simulink model "Basic_cosimulation_circuit"  (R2021b)
settings: Solver=ode4  StartTime=0.0  StopTime=inf  FixedStep=Ts  RelTol=1e-3  EnableMultiTasking=on
PostLoadFcn:
  | %
  | % Script for validation of swtiching model design with it's respective
  | % average model.
  | %
  | % Here it is presented the design of the inverter to the 6 kW Fuel Cell
  | % model.
  | 
  | %%% Initialization %%%
  | 
  | 
  | % ------------------------------------- %
  | % ---------- Inverter Design ---------- %
  | % ------------------------------------- %
  | 
  | %%%% Nominal Parameters %%%%
  | 
  | Pnom = 50e3;                                        % Nominal Power
  | Vdc = 400;                                          % DC Voltage - Boost
  | m = 0.6;                                            % Modulation Index
  | Vnom_peak = m*Vdc/2;                                % Peak Voltage
  | Vnom_rms = Vnom_peak/sqrt(2);                       % Rms Voltage
  | FP_min = 0.9;                                       % For Reactive Power
  |                                                     % Compensation
  | Snom = Pnom/FP_min;                                 % Apparent Power
  | Irms = Pnom/(sqrt(3)*Vnom_rms);                     % Rms Curren
  | Inom_peak = Irms*sqrt(2);                           % Peak Current
  | Zbase = Vnom_peak/Inom_peak;                        % Base Impedance
  | f = 60;                                             % Nominal Frequency
  | wnom = 2*pi*60;                                     % Angular Frequency
  | 
  | % ------------------------- %
  | % Inverter LC Filter Design %
  | % ------------------------- %
  | 
  | fsw_inv = 96*60;                                    % Switching Frequency must be a multiple of the nominal frequency
  |                                                      % for proper operation of the Artemis Block
  | ripple_inv = 0.03;
  | L_inv = ((Vdc/2)-Vnom_peak)*(1/fsw_inv)/(ripple_inv*Inom_peak);
  | 
  | % - Capacitor
  | fres = 420;                                         % Filters Ressonant Frequency
  | 
  | Cf = 1/(4*L_inv*(pi^2)*(fres^2));                % Filter Capacitor
  | Rf = 1/(wnom*Cf*50);                                % Damping Resistor
  | 
  | % --- Sample Time --- %
  | 
  | Tsw = 0.00050;
  | Ts = Tsw/10;
  | 
  | % ---------------------- %
  | % Current Control Design %
  | % ---------------------- %
  | 
  | Ron = 0.001;                                        % IGBT Resistance
  | tau_i = 1e-3;                                       % Responde Time
  | kp_current = L_inv/tau_i;                           % PI Proportional Gain
  | ki_current = (Ron)/tau_i;                           % PI Integral Gain
  | 
  | decouple = (wnom*L_inv);                            % Decoupling Gain
InitFcn:
  | %
  | % Script for validation of swtiching model design with it's respective
  | % average model.
  | %
  | % Here it is presented the design of the inverter to the 6 kW Fuel Cell
  | % model.
  | 
  | %%% Initialization %%%
  | 
  | 
  | % ------------------------------------- %
  | % ---------- Inverter Design ---------- %
  | % ------------------------------------- %
  | 
  | %%%% Nominal Parameters %%%%
  | 
  | Pnom = 50e3;                                        % Nominal Power
  | Vdc = 400;                                          % DC Voltage - Boost
  | m = 0.6;                                            % Modulation Index
  | Vnom_peak = m*Vdc/2;                                % Peak Voltage
  | Vnom_rms = Vnom_peak/sqrt(2);                       % Rms Voltage
  | FP_min = 0.9;                                       % For Reactive Power
  |                                                     % Compensation
  | Snom = Pnom/FP_min;                                 % Apparent Power
  | Irms = Pnom/(sqrt(3)*Vnom_rms);                     % Rms Curren
  | Inom_peak = Irms*sqrt(2);                           % Peak Current
  | Zbase = Vnom_peak/Inom_peak;                        % Base Impedance
  | f = 60;                                             % Nominal Frequency
  | wnom = 2*pi*60;                                     % Angular Frequency
  | 
  | % ------------------------- %
  | % Inverter LC Filter Design %
  | % ------------------------- %
  | 
  | fsw_inv = 96*60;                                    % Switching Frequency must be a multiple of the nominal frequency
  |                                                      % for proper operation of the Artemis Block
  | ripple_inv = 0.03;
  | L_inv = ((Vdc/2)-Vnom_peak)*(1/fsw_inv)/(ripple_inv*Inom_peak);
  | 
  | % - Capacitor
  | fres = 420;                                         % Filters Ressonant Frequency
  | 
  | Cf = 1/(4*L_inv*(pi^2)*(fres^2));                % Filter Capacitor
  | Rf = 1/(wnom*Cf*50);                                % Damping Resistor
  | 
  | % --- Sample Time --- %
  | 
  | Tsw = 0.00050;
  | Ts = Tsw/10;
  | 
  | % ---------------------- %
  | % Current Control Design %
  | % ---------------------- %
  | 
  | Ron = 0.001;                                        % IGBT Resistance
  | tau_i = 1e-3;                                       % Responde Time
  | kp_current = L_inv/tau_i;                           % PI Proportional Gain
  | ki_current = (Ron)/tau_i;                           % PI Integral Gain
  | 
  | decouple = (wnom*L_inv);                            % Decoupling Gain
undefined symbols (not defined in the file or in its folder): D1, Delta, DiscIntNeverNeededParam, IP, j, ph, sps, UDP
libraries: spsCurrentMeasurementLib x25, spsControlledVoltageSourceLib x21, rtlab x18, spsGroundLib x13, spsThreePhaseSeriesRLCBranchLib x13, spsControlledCurrentSourceLib x11, spsVoltageMeasurementLib x10, simulink x8, rteventslib x8, powerlib_meascontrol x7, spsThreePhaseVIMeasurementLib x4, ssn_inverter_model x4
(part 3 of 5)

== system Basic_cosimulation_circuit/SM_Master/Circuit_ITM_Source_DP_SFA/Phasor_to_Time_Domain_SFA ==
  Dynamic_Phasor : Inport
  Complex to Real-Imag4 : ComplexToRealImag
  Constant : Constant  Value=offset
  Demux : Demux  Outputs=3
  Demux1 : Demux  Outputs=2
  Gain : Gain  Gain=pi/180
  Gain3 : Gain  Gain=2*pi
  Gain4 : Gain  Gain=j*1
  Integrator : Integrator
  Magnitude-Angle to Complex : MagnitudeAngleToComplex
  Math Function : Math  SaturateOnIntegerOverflow=on
  Product : Product
  Real-Imag to Complex : RealImagToComplex
  Terminator : Terminator
  A : Outport
  B : Outport  Port=2
  C : Outport  Port=3
  wires:
  Demux/2 -> B/1
  Math Function/1 -> Product/2
  Gain4/1 -> Math Function/1
  Constant/1 -> Gain3/1
  Integrator/1 -> Gain4/1
  Dynamic_Phasor/1 -> Demux1/1
  Demux/1 -> A/1
  Product/1 -> Complex to Real-Imag4/1
  Gain3/1 -> Integrator/1
  Demux/3 -> C/1
  Complex to Real-Imag4/2 -> Terminator/1
  Complex to Real-Imag4/1 -> Demux/1
  Demux1/1 -> Real-Imag to Complex/1, Magnitude-Angle to Complex/1
  Demux1/2 -> Real-Imag to Complex/2, Gain/1
  Gain/1 -> Magnitude-Angle to Complex/2
  Real-Imag to Complex/1 -> Product/1

== system Basic_cosimulation_circuit/SM_Master/Circuit_ITM_Source_DP_SFA/Three-Phase Controlled Y-Connected Current Source ==
  Ia : Inport
  Ib : Inport  Port=2
  Ic : Inport  Port=3
  Controlled Current Source : spsControlledCurrentSourceLib/Controlled Current Source  Initialize=on  Source_Type=AC  Amplitude=0  Phase=0  Frequency=0  Measurements=None
  Controlled Current Source1 : spsControlledCurrentSourceLib/Controlled Current Source  Initialize=on  Source_Type=AC  Amplitude=0  Phase=0  Frequency=0  Measurements=None
  Controlled Current Source2 : spsControlledCurrentSourceLib/Controlled Current Source  Initialize=on  Source_Type=AC  Amplitude=0  Phase=0  Frequency=0  Measurements=None
  Ground1 : spsGroundLib/Ground  LConnTagsString=a
  A : PMIOPort  Side=Left
  B : PMIOPort  Port=2  Side=Left
  C : PMIOPort  Port=3  Side=Left
  wires:
  Ia/1 -> Controlled Current Source/1
  Ic/1 -> Controlled Current Source2/1
  Ib/1 -> Controlled Current Source1/1
  connections:
  Controlled Current Source/RConn1 -- Controlled Current Source2/RConn1 -- Ground1/LConn1 -- Controlled Current Source1/RConn1
  C/RConn1 -- Controlled Current Source2/LConn1
  B/RConn1 -- Controlled Current Source1/LConn1
  Controlled Current Source/LConn1 -- A/RConn1

== system Basic_cosimulation_circuit/SM_Master/Circuit_ITM_Source_DP_SFA/Time_Domain_To_Phasor_SFA ==
  EMT : Inport
  Complex to Magnitude-Angle : ComplexToMagnitudeAngle
  Complex to Magnitude-Angle1 : ComplexToMagnitudeAngle  Commented=on
  Complex to Real-Imag : ComplexToRealImag  Commented=on
  Complex to Real-Imag1 : ComplexToRealImag
  Constant : Constant  Value=offset
  Gain : Gain  Gain=j*(1/sqrt(3))*[0 1 -1; -1 0 1; 1 -1 0]  Multiplication=Matrix(K*u)
  Gain1 : Gain  Gain=180/pi
  Gain2 : Gain  Commented=on  Gain=j*(1/sqrt(3))*[0 1 -1; -1 0 1; 1 -1 0]  Multiplication=Matrix(K*u)
  Gain3 : Gain  Gain=-2*pi
  Gain4 : Gain  Gain=j*1
  Gain5 : Gain  Commented=on  Gain=180/pi
  Integrator : Integrator
  Math Function : Math  SaturateOnIntegerOverflow=on
  Mux1 : Mux  Inputs=2
  Mux2 : Mux  Commented=on  Inputs=2
  Mux3 : Mux  Inputs=2
  Phase/ Frequency Offset7 : commrflib2/Phase// Frequency Offset  Commented=on  phaseOffset=0  freqPort=off  freqOffset=-60
  Product : Product
  Scope : Scope
  Scope1 : Scope
  Scope2 : Scope  Commented=on  NumInputPorts=2
  Scope3 : Scope  Commented=on
  Scope4 : Scope  Commented=on
  Scope5 : Scope  Commented=on  NumInputPorts=2
  Scope6 : Scope
  Sum1 : Sum  Inputs=+|+
  Sum2 : Sum  Commented=on  Inputs=|++
  Dynamic_Phasor : Outport
  wires:
  Gain3/1 -> Integrator/1
  Sum1/1 -> Product/1
  Constant/1 -> Gain3/1
  Complex to Magnitude-Angle/1 -> Scope1/1, Mux1/1
  Gain/1 -> Sum1/1
  Gain1/1 -> Scope/1, Mux1/2
  Integrator/1 -> Gain4/1
  Math Function/1 -> Product/2
  Product/1 -> Complex to Real-Imag1/1, Complex to Magnitude-Angle/1
  Gain4/1 -> Math Function/1
  Complex to Magnitude-Angle/2 -> Gain1/1
  Gain2/1 -> Sum2/1
  Sum2/1 -> Scope2/2, Phase/ Frequency Offset7/1
  EMT/1 -> Sum1/2, Gain/1, Sum2/2, Scope2/1, Gain2/1
  Complex to Magnitude-Angle1/2 -> Gain5/1
  Phase/ Frequency Offset7/1 -> Complex to Real-Imag/1, Complex to Magnitude-Angle1/1
  Complex to Magnitude-Angle1/1 -> Scope4/1, Mux2/1
  Gain5/1 -> Scope3/1, Mux2/2
  Mux2/1 -> ?
  Complex to Real-Imag/2 -> Scope5/2
  Complex to Real-Imag/1 -> Scope5/1
  Complex to Real-Imag1/1 -> Mux3/1
  Complex to Real-Imag1/2 -> Mux3/2
  Mux3/1 -> Dynamic_Phasor/1, Scope6/1

== system Basic_cosimulation_circuit/SM_Master/Original Circuit/Control ==
  note: Control
  note: Transformation
  note: 3 Wire and PLL
  Vline : Inport
  Iabc : Inport  Port=2
  Deblock_inv : Inport  Port=3
  PQ_ref : Inport  Port=4
  Current Control : Subsystem
      settings: PortSchema="{\"entries\":[{\"content\":{\"sides\":[{\"content\":{\"connectorIds\":[\"In1\",\"In2\",\"In3\",\"In4\"]},\"type\":\"ConnectorPlacement.EquallySpacedRectSide\",\"uuid\":\"45a39461-35bf-48e0-8374-0f28be422fe8\"},{\"content\":{\"connectorIds\":[\"Out1\"],\"side\":\"RIGHT\"},\"type\":\"ConnectorPlacement.EquallySpacedRectSide\",\"uuid\":\"af171a1a-fd9b-46cd-ac56-6e4044580109\"},{\"content\":{\"connectorIds\":[\"In5\"],\"side\":\"TOP\"},\"type\":\"ConnectorPlacement.EquallySpacedRectSide\",\"uuid\":\"ea73d2ad-6043-4637-ba6c-414a87cf6777\"},{\"content\":{\"connectorIds\":[],\"side\":\"HIDDEN\"},\"type\":\"ConnectorPlacement.EquallySpacedRectSide\",\"uuid\":\"ed240fd2-007a-443e-85e9-b2acea2870c2\"}]},\"type\":\"ConnectorPlacement.EquallySpacedConnector\",\"uuid\":\"aa40401b-6e13-445e-a9b0-89ce19fbc40c\"}],\"packageUris\":[\"http://schema.mathworks.com/mf0/Connector/R2020b\"],\"version\":\"1.0\"}"
  Currents : Scope  NumInputPorts=2
  Demux : Demux  Outputs=2
  Demux1 : Demux  Outputs=2
  Meas_3_Wire : Subsystem
  Modulation : Scope
  Mux1 : Mux
  Mux2 : Mux  Inputs=2
  PQ Measure : Scope
  Park_Transformation : Subsystem
  Park_Transformation1 : Subsystem
  Power Control : Subsystem
      settings: PortSchema="{\"entries\":[{\"content\":{\"sides\":[{\"content\":{\"connectorIds\":[\"In1\"]},\"type\":\"ConnectorPlacement.EquallySpacedRectSide\",\"uuid\":\"974d39f2-3edd-4b06-9531-29f32c88933a\"},{\"content\":{\"connectorIds\":[\"Out1\"],\"side\":\"RIGHT\"},\"type\":\"ConnectorPlacement.EquallySpacedRectSide\",\"uuid\":\"24d62c8a-c61a-462a-84f0-1f0276c6dbaa\"},{\"content\":{\"connectorIds\":[],\"side\":\"TOP\"},\"type\":\"ConnectorPlacement.EquallySpacedRectSide\",\"uuid\":\"5ada6b1b-08a4-4e4d-9a20-cc19768e3a35\"},{\"content\":{\"connectorIds\":[\"In2\",\"In3\"],\"side\":\"BOTTOM\"},\"type\":\"ConnectorPlacement.EquallySpacedRectSide\",\"uuid\":\"aac35657-a4cf-4c82-a962-be637b231177\"},{\"content\":{\"connectorIds\":[],\"side\":\"HIDDEN\"},\"type\":\"ConnectorPlacement.EquallySpacedRectSide\",\"uuid\":\"6c2f95fb-9c8c-4eee-ad47-c57a643c3198\"}]},\"type\":\"ConnectorPlacement.EquallySpacedConnector\",\"uuid\":\"4f1b2c82-b884-470a-8be3-e486ca1ee764\"}],\"packageUris\":[\"http://schema.mathworks.com/mf0/Connector/R2020b\"],\"version\":\"1.0\"}"
  Power Measurement (Three-Phase) : eePowerMeasurement/Power Measurement (Three-Phase)  LabelModeActiveChoice=Continuous  F=60  K=[0 1 2 3]  Seq=Positive  Ts=0
      settings: SourceProductBaseCode=PS
  Product2 : Product
  SRF_PLL : Subsystem
  Saturation : Saturate  UpperLimit=1.1  LowerLimit=-1.1
  Terminator : Terminator
  Voltages : Scope  NumInputPorts=2
  Mabc : Outport
  Measures : Outport  Port=2
  wires:
  SRF_PLL/1(Phase) -> [phase_pll]
  Park_Transformation/1(DQ) -> Currents/2, [Idq]
  [Vabc] -> SRF_PLL/1(Vabc)
  [Vabc] -> Voltages/1, Park_Transformation1/1(ABC)
  Park_Transformation1/1(DQ) -> Voltages/2, Demux1/1, [Vdq]
  [phase_pll] -> Park_Transformation1/2(Phase)
  Saturation/1 -> Mabc/1, Modulation/1
  [dblk] -> Product2/2
  Iabc/1 -> Park_Transformation/1(ABC), Currents/1, [Iabc]
  Meas_3_Wire/1(ABC) -> [Vabc]
  Product2/1 -> Saturation/1
  Vline/1 -> Demux/1
  Demux/1 -> Meas_3_Wire/1(AB)
  Demux/2 -> Meas_3_Wire/2(BC)
  Mux1/1 -> Measures/1
  [Vdq] -> Mux1/3
  [Iabc] -> Mux1/2
  [Vabc] -> Mux1/4
  [Idq] -> Mux1/1
  Deblock_inv/1 -> [dblk], Current Control/1(Deblock)
  Current Control/1(modulation) -> Product2/1
  [Idq] -> Current Control/3(Idq)
  [Vdq] -> Current Control/4(Vdq)
  [phase_pll] -> Current Control/5(Phase)
  [phase_pll] -> Park_Transformation/2(Phase)
  Demux1/2 -> Terminator/1
  Demux1/1 -> [Vd]
  PQ_ref/1 -> Power Control/1(PQ_ref)
  [Vd] -> Power Control/2(Vd)
  [dblk] -> Power Control/3(Dblk)
  Power Control/1(Out1) -> Current Control/2(Idq_ref)
  [Vabc] -> Power Measurement (Three-Phase)/1
  [Iabc] -> Power Measurement (Three-Phase)/2
  Power Measurement (Three-Phase)/2 -> Mux2/2
  Power Measurement (Three-Phase)/1 -> Mux2/1
  Mux2/1 -> PQ Measure/1

== system Basic_cosimulation_circuit/SM_Master/Original Circuit/PWM ==
  Uabc_ref : Inport
  Constant10 : Constant  Value=2
  Constant11 : Constant  Value=fsw_inv
  Constant9 : Constant
  Demux8 : Demux  Outputs=3
  Divide7 : Product  Inputs=*/
  Divide8 : Product  Inputs=*/
  Divide9 : Product  Inputs=*/
  Mux11 : Mux  Inputs=3
  Mux12 : Mux  Inputs=2
  RTE Conversion1 : rteventslib/Signal Attributes/RTE Conversion  inputdatatype=RTE Boolean  outputdatatype=Double  compensation=Enabled  nbMaxEvents=4  sampleTime=Ts
  RTE SPWM1 : rteventslib/Sources/RTE SPWM  NumberPhases=3-ph  CenterAlignmentMode=On  MaxFreq=inf  MinFreq=0  EnablingPort=off  ComplementaryMode=on  SpaceVector=off  RiseTimeDelay=0  MaxEvents=4  SampleTime=Ts
  Scope : Scope
  Scope8 : Scope
  Selector1 : Selector  InputPortWidth=6  IndexOptions=Index vector (dialog)  Indices=[1 4 2 5 3 6]  OutputSizes=1
  Sum16 : Sum  Inputs=|++
  Sum17 : Sum  Inputs=|++
  Sum18 : Sum  Inputs=|++
  Uref : Outport  VectorParamsAs1DForOutWhenUnconnected=off
  wires:
  Uabc_ref/1 -> Demux8/1, Scope/1
  RTE SPWM1/1 -> Mux12/1
  Constant9/1 -> Sum18/2, Sum17/2, Sum16/2
  Selector1/1 -> Uref/1
  Constant11/1 -> RTE SPWM1/1
  Sum16/1 -> Divide7/1
  Constant10/1 -> Divide9/2, Divide8/2, Divide7/2
  Sum17/1 -> Divide8/1
  Divide9/1 -> Mux11/3
  RTE SPWM1/2 -> Mux12/2
  Demux8/2 -> Sum17/1
  Divide8/1 -> Mux11/2
  Sum18/1 -> Divide9/1
  Mux11/1 -> RTE SPWM1/2, Scope8/1
  Divide7/1 -> Mux11/1
  Demux8/1 -> Sum16/1
  Demux8/3 -> Sum18/1
  Mux12/1 -> RTE Conversion1/1
  RTE Conversion1/1 -> Selector1/1

== system Basic_cosimulation_circuit/SM_Master/Original_Circuit/Controllable Voltage Source  ==
  Amplitude [V] : Inport
  Phase [Deg] : Inport  Port=2
  Frequency [Hz] : Inport  Port=3
  Constant1 : Constant  Value=2*pi/3
  Controlled Voltage Source3 : spsControlledVoltageSourceLib/Controlled Voltage Source  Initialize=on  Source_Type=AC  Amplitude=0  Phase=0  Frequency=0  Measurements=None
  Controlled Voltage Source4 : spsControlledVoltageSourceLib/Controlled Voltage Source  Initialize=on  Source_Type=AC  Amplitude=0  Phase=0  Frequency=0  Measurements=None
  Controlled Voltage Source5 : spsControlledVoltageSourceLib/Controlled Voltage Source  Initialize=on  Source_Type=AC  Amplitude=0  Phase=0  Frequency=0  Measurements=None
  Cos : Trigonometry  Operator=cos
  Cos1 : Trigonometry  Operator=cos
  Cos2 : Trigonometry  Operator=cos
  Gain : Gain  Gain=2*pi
  Gain1 : Gain  Gain=pi/180
  Ground5 : spsGroundLib/Ground  LConnTagsString=a
  Integrator : Integrator  WrapState=on  WrappedStateUpperValue=2*pi  WrappedStateLowerValue=0
  Product : Product
  Product1 : Product
  Product2 : Product
  Sum : Sum  Inputs=++-
  Sum1 : Sum  Inputs=+++
  Sum2 : Sum  Inputs=|++
  A : PMIOPort  Side=Right
  B : PMIOPort  Port=2  Side=Right
  C : PMIOPort  Port=3  Side=Right
  wires:
  Sum/1 -> Cos1/1
  Amplitude [V]/1 -> Product2/1, Product1/1, Product/1
  Integrator/1 -> [phase]
  Gain/1 -> Integrator/1
  Phase [Deg]/1 -> Gain1/1
  Constant1/1 -> Sum/3, Sum1/2
  Sum2/1 -> Cos/1
  Product/1 -> Controlled Voltage Source3/1
  Cos/1 -> Product/2
  [phase] -> Sum2/1, Sum/2, Sum1/1
  Product1/1 -> Controlled Voltage Source4/1
  Product2/1 -> Controlled Voltage Source5/1
  Sum1/1 -> Cos2/1
  Cos1/1 -> Product1/2
  Cos2/1 -> Product2/2
  Frequency [Hz]/1 -> [freq_ref], Gain/1
  Gain1/1 -> Sum1/3, Sum/1, Sum2/2
  connections:
  Controlled Voltage Source4/RConn1 -- B/RConn1
  Controlled Voltage Source3/RConn1 -- A/RConn1
  Controlled Voltage Source5/RConn1 -- C/RConn1
  Controlled Voltage Source4/LConn1 -- Ground5/LConn1 -- Controlled Voltage Source5/LConn1 -- Controlled Voltage Source3/LConn1

== system Basic_cosimulation_circuit/SM_Master/VSC_ITM_Average_Moving_Window/Control ==
  note: Control
  note: Transformation
  note: 3 Wire and PLL
  Vline : Inport
  Iabc : Inport  Port=2
  Deblock_inv : Inport  Port=3
  PQ_ref : Inport  Port=4
  Current Control : Subsystem
      settings: PortSchema="{\"entries\":[{\"content\":{\"sides\":[{\"content\":{\"connectorIds\":[\"In1\",\"In2\",\"In3\",\"In4\"]},\"type\":\"ConnectorPlacement.EquallySpacedRectSide\",\"uuid\":\"45a39461-35bf-48e0-8374-0f28be422fe8\"},{\"content\":{\"connectorIds\":[\"Out1\"],\"side\":\"RIGHT\"},\"type\":\"ConnectorPlacement.EquallySpacedRectSide\",\"uuid\":\"af171a1a-fd9b-46cd-ac56-6e4044580109\"},{\"content\":{\"connectorIds\":[\"In5\"],\"side\":\"TOP\"},\"type\":\"ConnectorPlacement.EquallySpacedRectSide\",\"uuid\":\"ea73d2ad-6043-4637-ba6c-414a87cf6777\"},{\"content\":{\"connectorIds\":[],\"side\":\"HIDDEN\"},\"type\":\"ConnectorPlacement.EquallySpacedRectSide\",\"uuid\":\"ed240fd2-007a-443e-85e9-b2acea2870c2\"}]},\"type\":\"ConnectorPlacement.EquallySpacedConnector\",\"uuid\":\"aa40401b-6e13-445e-a9b0-89ce19fbc40c\"}],\"packageUris\":[\"http://schema.mathworks.com/mf0/Connector/R2020b\"],\"version\":\"1.0\"}"
  Currents : Scope  NumInputPorts=2
  Demux : Demux  Outputs=2
  Demux1 : Demux  Outputs=2
  Meas_3_Wire : Subsystem
  Modulation : Scope  Commented=on
  Mux1 : Mux  Inputs=5
  Mux2 : Mux  Inputs=2
  Park_Transformation : Subsystem
  Park_Transformation1 : Subsystem
  Power Control : Subsystem
      settings: PortSchema="{\"entries\":[{\"content\":{\"sides\":[{\"content\":{\"connectorIds\":[\"In1\"]},\"type\":\"ConnectorPlacement.EquallySpacedRectSide\",\"uuid\":\"974d39f2-3edd-4b06-9531-29f32c88933a\"},{\"content\":{\"connectorIds\":[\"Out1\"],\"side\":\"RIGHT\"},\"type\":\"ConnectorPlacement.EquallySpacedRectSide\",\"uuid\":\"24d62c8a-c61a-462a-84f0-1f0276c6dbaa\"},{\"content\":{\"connectorIds\":[],\"side\":\"TOP\"},\"type\":\"ConnectorPlacement.EquallySpacedRectSide\",\"uuid\":\"5ada6b1b-08a4-4e4d-9a20-cc19768e3a35\"},{\"content\":{\"connectorIds\":[\"In2\",\"In3\"],\"side\":\"BOTTOM\"},\"type\":\"ConnectorPlacement.EquallySpacedRectSide\",\"uuid\":\"aac35657-a4cf-4c82-a962-be637b231177\"},{\"content\":{\"connectorIds\":[],\"side\":\"HIDDEN\"},\"type\":\"ConnectorPlacement.EquallySpacedRectSide\",\"uuid\":\"6c2f95fb-9c8c-4eee-ad47-c57a643c3198\"}]},\"type\":\"ConnectorPlacement.EquallySpacedConnector\",\"uuid\":\"4f1b2c82-b884-470a-8be3-e486ca1ee764\"}],\"packageUris\":[\"http://schema.mathworks.com/mf0/Connector/R2020b\"],\"version\":\"1.0\"}"
  Power Measurement (Three-Phase) : eePowerMeasurement/Power Measurement (Three-Phase)  LabelModeActiveChoice=Discrete  F=60  K=[1]  Seq=Positive  Ts=Ts
      settings: SourceProductBaseCode=PS
  Product2 : Product
  SRF_PLL : Subsystem
  Saturation : Saturate  UpperLimit=1.1  LowerLimit=-1.1
  Terminator : Terminator
  Voltages : Scope  Commented=on  NumInputPorts=2
  Mabc : Outport
  Measures : Outport  Port=2
  Vabc : Outport  Port=3
  wires:
  SRF_PLL/1(Phase) -> [phase_pll]
  Park_Transformation/1(DQ) -> Currents/2, [Idq]
  [Vabc] -> SRF_PLL/1(Vabc)
  [Vabc] -> Voltages/1, Park_Transformation1/1(ABC)
  Park_Transformation1/1(DQ) -> Voltages/2, Demux1/1, [Vdq]
  [phase_pll] -> Park_Transformation1/2(Phase)
  Saturation/1 -> Mabc/1, Modulation/1
  [dblk] -> Product2/2
  Iabc/1 -> Park_Transformation/1(ABC), Currents/1, [Iabc]
  Meas_3_Wire/1(ABC) -> [Vabc]
  Product2/1 -> Saturation/1
  Vline/1 -> Demux/1
  Demux/1 -> Meas_3_Wire/1(AB)
  Demux/2 -> Meas_3_Wire/2(BC)
  Mux1/1 -> Measures/1
  [Vdq] -> Mux1/3
  [Iabc] -> Mux1/2
  [Vabc] -> Mux1/4, Vabc/1
  [Idq] -> Mux1/1
  Deblock_inv/1 -> [dblk], Current Control/1(Deblock)
  Current Control/1(modulation) -> Product2/1
  [Idq] -> Current Control/3(Idq)
  [Vdq] -> Current Control/4(Vdq)
  [phase_pll] -> Current Control/5(Phase)
  [phase_pll] -> Park_Transformation/2(Phase)
  Demux1/2 -> Terminator/1
  Demux1/1 -> [Vd]
  PQ_ref/1 -> Power Control/1(PQ_ref)
  [Vd] -> Power Control/2(Vd)
  [dblk] -> Power Control/3(Dblk)
  Power Control/1(Out1) -> Current Control/2(Idq_ref)
  [Vabc] -> Power Measurement (Three-Phase)/1
  [Iabc] -> Power Measurement (Three-Phase)/2
  Power Measurement (Three-Phase)/2 -> Mux2/2
  Power Measurement (Three-Phase)/1 -> Mux2/1
  Mux2/1 -> [pq_meas]
  [pq_meas] -> Mux1/5

== system Basic_cosimulation_circuit/SM_Master/VSC_ITM_Average_Moving_Window/DP - > EMT ==
  Phasor_A : Inport
  Phasor_B : Inport  Port=2
  Phasor_C : Inport  Port=3
  Demux : Demux  Outputs=2
  Demux1 : Demux  Outputs=2
  Demux2 : Demux  Outputs=2
  Subsystem : Subsystem
  Subsystem1 : Subsystem
  Subsystem2 : Subsystem
  Sinal_A : Outport
  Sinal_B : Outport  Port=2
  Sinal_C : Outport  Port=3
  wires:
  Subsystem2/1(Out1) -> Sinal_C/1
  Subsystem1/1(Out1) -> Sinal_B/1
  Subsystem/1(Out1) -> Sinal_A/1
  Demux/1 -> Subsystem/1(In1)
  Demux/2 -> Subsystem/2(Input)
  Demux1/1 -> Subsystem1/1(In1)
  Demux1/2 -> Subsystem1/2(Input1)
  Demux2/1 -> Subsystem2/1(In1)
  Demux2/2 -> Subsystem2/2(Input2)
  Phasor_A/1 -> Demux/1
  Phasor_B/1 -> Demux1/1
  Phasor_C/1 -> Demux2/1

== system Basic_cosimulation_circuit/SM_Master/VSC_ITM_Average_Moving_Window/Dynamic Phasor coeficientes extraction ==
  EMT_Signal : Inport
  Demux : Demux  Outputs=3
  Fourier_A : powerlib_meascontrol/Measurements/Fourier  Freq=60  n=1  InInit=[1,0]  Ts=Ts
  Fourier_B : powerlib_meascontrol/Measurements/Fourier  Freq=60  n=1  InInit=[1,-120 ]  Ts=Ts
  Fourier_C : powerlib_meascontrol/Measurements/Fourier  Freq=60  n=1  InInit=[1,+120 ]  Ts=Ts
  Mux : Mux  Inputs=2
  Mux1 : Mux  Inputs=2
  Mux2 : Mux  Inputs=2
  deg->rad : Gain  Gain=pi/180  SaturateOnIntegerOverflow=on  OutDataTypeStr=Inherit: Same as input  ParamDataTypeStr=Inherit: Same as input
  deg->rad1 : Gain  Gain=pi/180  SaturateOnIntegerOverflow=on  OutDataTypeStr=Inherit: Same as input  ParamDataTypeStr=Inherit: Same as input
  deg->rad2 : Gain  Gain=pi/180  SaturateOnIntegerOverflow=on  OutDataTypeStr=Inherit: Same as input  ParamDataTypeStr=Inherit: Same as input
  Phasor_A : Outport
  Phasor_B : Outport  Port=2
  Phasor_C : Outport  Port=3
  wires:
  Demux/2 -> Fourier_B/1
  deg->rad1/1 -> Mux2/2
  Demux/3 -> Fourier_C/1
  Demux/1 -> Fourier_A/1
  Fourier_C/1 -> Mux1/1
  EMT_Signal/1 -> Demux/1
  Fourier_B/2 -> deg->rad1/1
  deg->rad2/1 -> Mux1/2
  Fourier_A/2 -> deg->rad/1
  Fourier_C/2 -> deg->rad2/1
  Fourier_A/1 -> Mux/1
  deg->rad/1 -> Mux/2
  Fourier_B/1 -> Mux2/1
  Mux/1 -> Phasor_A/1
  Mux2/1 -> Phasor_B/1
  Mux1/1 -> Phasor_C/1

== system Basic_cosimulation_circuit/SM_Master/VSC_ITM_Average_Moving_Window/PWM ==
  Uabc_ref : Inport
  Constant10 : Constant  Value=2
  Constant11 : Constant  Value=fsw_inv
  Constant9 : Constant
  Demux8 : Demux  Outputs=3
  Divide7 : Product  Inputs=*/
  Divide8 : Product  Inputs=*/
  Divide9 : Product  Inputs=*/
  Mux11 : Mux  Inputs=3
  Mux12 : Mux  Inputs=2
  RTE Conversion1 : rteventslib/Signal Attributes/RTE Conversion  inputdatatype=RTE Boolean  outputdatatype=Double  compensation=Enabled  nbMaxEvents=4  sampleTime=Ts
  RTE SPWM1 : rteventslib/Sources/RTE SPWM  NumberPhases=3-ph  CenterAlignmentMode=On  MaxFreq=inf  MinFreq=0  EnablingPort=off  ComplementaryMode=on  SpaceVector=off  RiseTimeDelay=0  MaxEvents=4  SampleTime=Ts
  Scope : Scope
  Scope8 : Scope
  Selector1 : Selector  InputPortWidth=6  IndexOptions=Index vector (dialog)  Indices=[1 4 2 5 3 6]  OutputSizes=1
  Sum16 : Sum  Inputs=|++
  Sum17 : Sum  Inputs=|++
  Sum18 : Sum  Inputs=|++
  Uref : Outport  VectorParamsAs1DForOutWhenUnconnected=off
  wires:
  Uabc_ref/1 -> Demux8/1, Scope/1
  RTE SPWM1/1 -> Mux12/1
  Constant9/1 -> Sum18/2, Sum17/2, Sum16/2
  Selector1/1 -> Uref/1
  Constant11/1 -> RTE SPWM1/1
  Sum16/1 -> Divide7/1
  Constant10/1 -> Divide9/2, Divide8/2, Divide7/2
  Sum17/1 -> Divide8/1
  Divide9/1 -> Mux11/3
  RTE SPWM1/2 -> Mux12/2
  Demux8/2 -> Sum17/1
  Divide8/1 -> Mux11/2
  Sum18/1 -> Divide9/1
  Mux11/1 -> RTE SPWM1/2, Scope8/1
  Divide7/1 -> Mux11/1
  Demux8/1 -> Sum16/1
  Demux8/3 -> Sum18/1
  Mux12/1 -> RTE Conversion1/1
  RTE Conversion1/1 -> Selector1/1

== system Basic_cosimulation_circuit/SM_Master/VSC_ITM_Average_Moving_Window/Three-Phase Controlled Y-Connected Voltage Source  ==
  Va : Inport
  Vb : Inport  Port=2
  Vc : Inport  Port=3
  Controlled Voltage Source : spsControlledVoltageSourceLib/Controlled Voltage Source  Initialize=off  Source_Type=AC  Amplitude=0  Phase=0  Frequency=0  Measurements=None
  Controlled Voltage Source1 : spsControlledVoltageSourceLib/Controlled Voltage Source  Initialize=off  Source_Type=AC  Amplitude=0  Phase=0  Frequency=0  Measurements=None
  Controlled Voltage Source2 : spsControlledVoltageSourceLib/Controlled Voltage Source  Initialize=off  Source_Type=AC  Amplitude=0  Phase=0  Frequency=0  Measurements=None
  Ground : spsGroundLib/Ground  LConnTagsString=a
  + : PMIOPort  Side=Right
  +1 : PMIOPort  Port=2  Side=Right
  +2 : PMIOPort  Port=3  Side=Right
  wires:
  Vb/1 -> Controlled Voltage Source1/1
  Va/1 -> Controlled Voltage Source/1
  Vc/1 -> Controlled Voltage Source2/1
  connections:
  Controlled Voltage Source/RConn1 -- +/RConn1
  Controlled Voltage Source1/RConn1 -- +1/RConn1
  Controlled Voltage Source2/RConn1 -- +2/RConn1
  Controlled Voltage Source2/LConn1 -- Controlled Voltage Source/LConn1 -- Controlled Voltage Source1/LConn1 -- Ground/LConn1

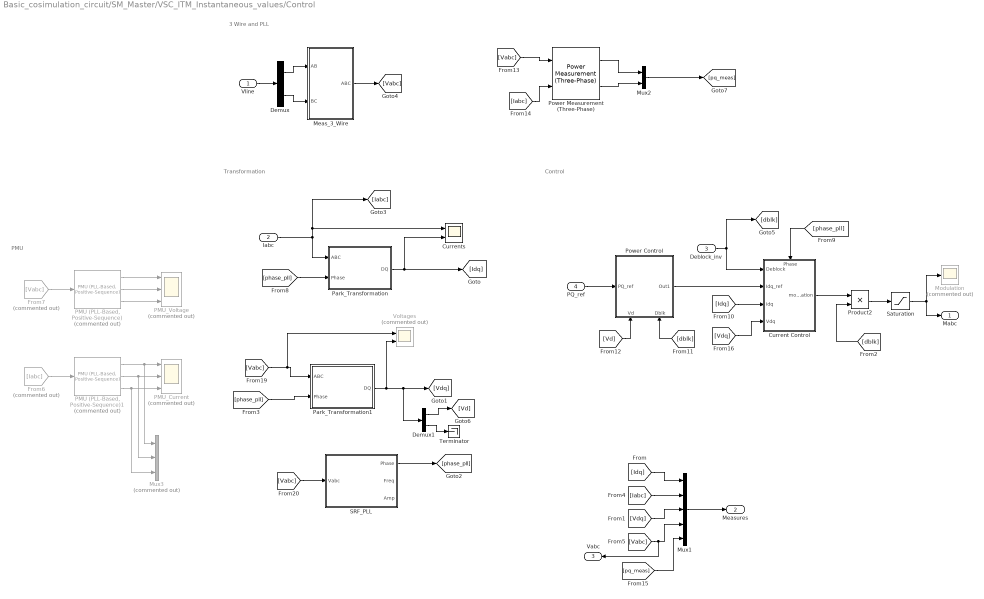
== system Basic_cosimulation_circuit/SM_Master/VSC_ITM_Instantaneous_values/Control ==
  note: PMU
  note: Control
  note: Transformation
  note: 3 Wire and PLL
  Vline : Inport
  Iabc : Inport  Port=2
  Deblock_inv : Inport  Port=3
  PQ_ref : Inport  Port=4
  Current Control : Subsystem
      settings: PortSchema="{\"entries\":[{\"content\":{\"sides\":[{\"content\":{\"connectorIds\":[\"In1\",\"In2\",\"In3\",\"In4\"]},\"type\":\"ConnectorPlacement.EquallySpacedRectSide\",\"uuid\":\"45a39461-35bf-48e0-8374-0f28be422fe8\"},{\"content\":{\"connectorIds\":[\"Out1\"],\"side\":\"RIGHT\"},\"type\":\"ConnectorPlacement.EquallySpacedRectSide\",\"uuid\":\"af171a1a-fd9b-46cd-ac56-6e4044580109\"},{\"content\":{\"connectorIds\":[\"In5\"],\"side\":\"TOP\"},\"type\":\"ConnectorPlacement.EquallySpacedRectSide\",\"uuid\":\"ea73d2ad-6043-4637-ba6c-414a87cf6777\"},{\"content\":{\"connectorIds\":[],\"side\":\"HIDDEN\"},\"type\":\"ConnectorPlacement.EquallySpacedRectSide\",\"uuid\":\"ed240fd2-007a-443e-85e9-b2acea2870c2\"}]},\"type\":\"ConnectorPlacement.EquallySpacedConnector\",\"uuid\":\"aa40401b-6e13-445e-a9b0-89ce19fbc40c\"}],\"packageUris\":[\"http://schema.mathworks.com/mf0/Connector/R2020b\"],\"version\":\"1.0\"}"
  Currents : Scope  NumInputPorts=2
  Demux : Demux  Outputs=2
  Demux1 : Demux  Outputs=2
  From6 : From  Commented=on  GotoTag=Iabc
  From7 : From  Commented=on  GotoTag=Vabc
  Meas_3_Wire : Subsystem
  Modulation : Scope  Commented=on
  Mux1 : Mux  Inputs=5
  Mux2 : Mux  Inputs=2
  Mux3 : Mux  Commented=on  Inputs=3
  "PMU (PLL-Based, Positive-Sequence)" : powerlib_meascontrol/Measurements/PMU (PLL-Based, Positive-Sequence)  Commented=on  nominalFrequency=60  samplingRate=48  reportingFactor=1
      settings: SourceProductBaseCode=PS
  "PMU (PLL-Based, Positive-Sequence)1" : powerlib_meascontrol/Measurements/PMU (PLL-Based, Positive-Sequence)  Commented=on  nominalFrequency=60  samplingRate=48  reportingFactor=1
      settings: SourceProductBaseCode=PS
  PMU_Current : Scope  Commented=on  NumInputPorts=3
  PMU_Voltage : Scope  Commented=on  NumInputPorts=3
  Park_Transformation : Subsystem
  Park_Transformation1 : Subsystem
  Power Control : Subsystem
      settings: PortSchema="{\"entries\":[{\"content\":{\"sides\":[{\"content\":{\"connectorIds\":[\"In1\"]},\"type\":\"ConnectorPlacement.EquallySpacedRectSide\",\"uuid\":\"974d39f2-3edd-4b06-9531-29f32c88933a\"},{\"content\":{\"connectorIds\":[\"Out1\"],\"side\":\"RIGHT\"},\"type\":\"ConnectorPlacement.EquallySpacedRectSide\",\"uuid\":\"24d62c8a-c61a-462a-84f0-1f0276c6dbaa\"},{\"content\":{\"connectorIds\":[],\"side\":\"TOP\"},\"type\":\"ConnectorPlacement.EquallySpacedRectSide\",\"uuid\":\"5ada6b1b-08a4-4e4d-9a20-cc19768e3a35\"},{\"content\":{\"connectorIds\":[\"In2\",\"In3\"],\"side\":\"BOTTOM\"},\"type\":\"ConnectorPlacement.EquallySpacedRectSide\",\"uuid\":\"aac35657-a4cf-4c82-a962-be637b231177\"},{\"content\":{\"connectorIds\":[],\"side\":\"HIDDEN\"},\"type\":\"ConnectorPlacement.EquallySpacedRectSide\",\"uuid\":\"6c2f95fb-9c8c-4eee-ad47-c57a643c3198\"}]},\"type\":\"ConnectorPlacement.EquallySpacedConnector\",\"uuid\":\"4f1b2c82-b884-470a-8be3-e486ca1ee764\"}],\"packageUris\":[\"http://schema.mathworks.com/mf0/Connector/R2020b\"],\"version\":\"1.0\"}"
  Power Measurement (Three-Phase) : eePowerMeasurement/Power Measurement (Three-Phase)  LabelModeActiveChoice=Discrete  F=60  K=[1]  Seq=Positive  Ts=Ts
      settings: SourceProductBaseCode=PS
  Product2 : Product
  SRF_PLL : Subsystem
  Saturation : Saturate  UpperLimit=1.1  LowerLimit=-1.1
  Terminator : Terminator
  Voltages : Scope  Commented=on  NumInputPorts=2
  Mabc : Outport
  Measures : Outport  Port=2
  Vabc : Outport  Port=3
  wires:
  SRF_PLL/1(Phase) -> [phase_pll]
  Park_Transformation/1(DQ) -> Currents/2, [Idq]
  [Vabc] -> SRF_PLL/1(Vabc)
  [Vabc] -> Voltages/1, Park_Transformation1/1(ABC)
  Park_Transformation1/1(DQ) -> Voltages/2, Demux1/1, [Vdq]
  [phase_pll] -> Park_Transformation1/2(Phase)
  Saturation/1 -> Mabc/1, Modulation/1
  [dblk] -> Product2/2
  Iabc/1 -> Park_Transformation/1(ABC), Currents/1, [Iabc]
  Meas_3_Wire/1(ABC) -> [Vabc]
  Product2/1 -> Saturation/1
  Vline/1 -> Demux/1
  Demux/1 -> Meas_3_Wire/1(AB)
  Demux/2 -> Meas_3_Wire/2(BC)
  Mux1/1 -> Measures/1
  [Vdq] -> Mux1/3
  [Iabc] -> Mux1/2
  [Vabc] -> Mux1/4, Vabc/1
  [Idq] -> Mux1/1
  From7/1 -> "PMU (PLL-Based, Positive-Sequence)"/1
  From6/1 -> "PMU (PLL-Based, Positive-Sequence)1"/1
  "PMU (PLL-Based, Positive-Sequence)"/1 -> PMU_Voltage/1
  "PMU (PLL-Based, Positive-Sequence)"/2 -> PMU_Voltage/2
  "PMU (PLL-Based, Positive-Sequence)"/3 -> PMU_Voltage/3
  "PMU (PLL-Based, Positive-Sequence)1"/1 -> Mux3/1, PMU_Current/1
  "PMU (PLL-Based, Positive-Sequence)1"/2 -> Mux3/2, PMU_Current/2
  "PMU (PLL-Based, Positive-Sequence)1"/3 -> Mux3/3, PMU_Current/3
  Deblock_inv/1 -> [dblk], Current Control/1(Deblock)
  Current Control/1(modulation) -> Product2/1
  [Idq] -> Current Control/3(Idq)
  [Vdq] -> Current Control/4(Vdq)
  [phase_pll] -> Current Control/5(Phase)
  [phase_pll] -> Park_Transformation/2(Phase)
  Demux1/2 -> Terminator/1
  Demux1/1 -> [Vd]
  PQ_ref/1 -> Power Control/1(PQ_ref)
  [Vd] -> Power Control/2(Vd)
  [dblk] -> Power Control/3(Dblk)
  Power Control/1(Out1) -> Current Control/2(Idq_ref)
  [Vabc] -> Power Measurement (Three-Phase)/1
  [Iabc] -> Power Measurement (Three-Phase)/2
  Power Measurement (Three-Phase)/2 -> Mux2/2
  Power Measurement (Three-Phase)/1 -> Mux2/1
  Mux2/1 -> [pq_meas]
  [pq_meas] -> Mux1/5

== system Basic_cosimulation_circuit/SM_Master/VSC_ITM_Instantaneous_values/PWM ==
  Uabc_ref : Inport
  Constant10 : Constant  Value=2
  Constant11 : Constant  Value=fsw_inv
  Constant9 : Constant
  Demux8 : Demux  Outputs=3
  Divide7 : Product  Inputs=*/
  Divide8 : Product  Inputs=*/
  Divide9 : Product  Inputs=*/
  Mux11 : Mux  Inputs=3
  Mux12 : Mux  Inputs=2
  RTE Conversion1 : rteventslib/Signal Attributes/RTE Conversion  inputdatatype=RTE Boolean  outputdatatype=Double  compensation=Enabled  nbMaxEvents=4  sampleTime=Ts
  RTE SPWM1 : rteventslib/Sources/RTE SPWM  NumberPhases=3-ph  CenterAlignmentMode=On  MaxFreq=inf  MinFreq=0  EnablingPort=off  ComplementaryMode=on  SpaceVector=off  RiseTimeDelay=0  MaxEvents=4  SampleTime=Ts
  Scope : Scope
  Scope8 : Scope
  Selector1 : Selector  InputPortWidth=6  IndexOptions=Index vector (dialog)  Indices=[1 4 2 5 3 6]  OutputSizes=1
  Sum16 : Sum  Inputs=|++
  Sum17 : Sum  Inputs=|++
  Sum18 : Sum  Inputs=|++
  Uref : Outport  VectorParamsAs1DForOutWhenUnconnected=off
  wires:
  Uabc_ref/1 -> Demux8/1, Scope/1
  RTE SPWM1/1 -> Mux12/1
  Constant9/1 -> Sum18/2, Sum17/2, Sum16/2
  Selector1/1 -> Uref/1
  Constant11/1 -> RTE SPWM1/1
  Sum16/1 -> Divide7/1
  Constant10/1 -> Divide9/2, Divide8/2, Divide7/2
  Sum17/1 -> Divide8/1
  Divide9/1 -> Mux11/3
  RTE SPWM1/2 -> Mux12/2
  Demux8/2 -> Sum17/1
  Divide8/1 -> Mux11/2
  Sum18/1 -> Divide9/1
  Mux11/1 -> RTE SPWM1/2, Scope8/1
  Divide7/1 -> Mux11/1
  Demux8/1 -> Sum16/1
  Demux8/3 -> Sum18/1
  Mux12/1 -> RTE Conversion1/1
  RTE Conversion1/1 -> Selector1/1

== system Basic_cosimulation_circuit/SM_Master/VSC_ITM_Instantaneous_values/Three-Phase Controlled Y-Connected Voltage Source  ==
  Va : Inport
  Vb : Inport  Port=2
  Vc : Inport  Port=3
  Controlled Voltage Source : spsControlledVoltageSourceLib/Controlled Voltage Source  Initialize=off  Source_Type=AC  Amplitude=0  Phase=0  Frequency=0  Measurements=None
  Controlled Voltage Source1 : spsControlledVoltageSourceLib/Controlled Voltage Source  Initialize=off  Source_Type=AC  Amplitude=0  Phase=0  Frequency=0  Measurements=None
  Controlled Voltage Source2 : spsControlledVoltageSourceLib/Controlled Voltage Source  Initialize=off  Source_Type=AC  Amplitude=0  Phase=0  Frequency=0  Measurements=None
  Ground : spsGroundLib/Ground  LConnTagsString=a
  + : PMIOPort  Side=Right
  +1 : PMIOPort  Port=2  Side=Right
  +2 : PMIOPort  Port=3  Side=Right
  wires:
  Vb/1 -> Controlled Voltage Source1/1
  Va/1 -> Controlled Voltage Source/1
  Vc/1 -> Controlled Voltage Source2/1
  connections:
  Controlled Voltage Source/RConn1 -- +/RConn1
  Controlled Voltage Source1/RConn1 -- +1/RConn1
  Controlled Voltage Source2/RConn1 -- +2/RConn1
  Controlled Voltage Source2/LConn1 -- Controlled Voltage Source/LConn1 -- Controlled Voltage Source1/LConn1 -- Ground/LConn1

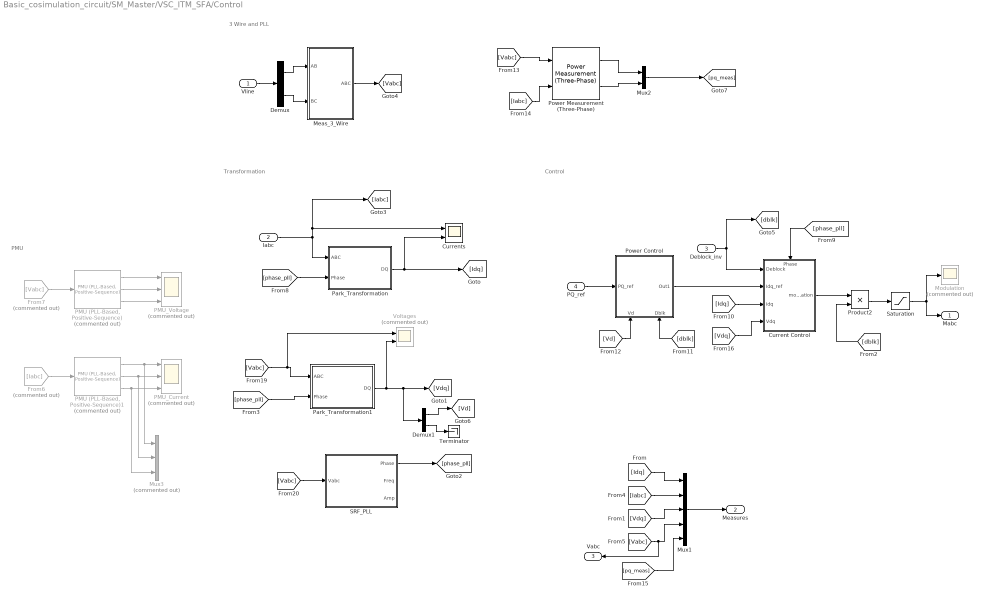
== system Basic_cosimulation_circuit/SM_Master/VSC_ITM_SFA/Control ==
  note: PMU
  note: Control
  note: Transformation
  note: 3 Wire and PLL
  Vline : Inport
  Iabc : Inport  Port=2
  Deblock_inv : Inport  Port=3
  PQ_ref : Inport  Port=4
  Current Control : Subsystem
      settings: PortSchema="{\"entries\":[{\"content\":{\"sides\":[{\"content\":{\"connectorIds\":[\"In1\",\"In2\",\"In3\",\"In4\"]},\"type\":\"ConnectorPlacement.EquallySpacedRectSide\",\"uuid\":\"45a39461-35bf-48e0-8374-0f28be422fe8\"},{\"content\":{\"connectorIds\":[\"Out1\"],\"side\":\"RIGHT\"},\"type\":\"ConnectorPlacement.EquallySpacedRectSide\",\"uuid\":\"af171a1a-fd9b-46cd-ac56-6e4044580109\"},{\"content\":{\"connectorIds\":[\"In5\"],\"side\":\"TOP\"},\"type\":\"ConnectorPlacement.EquallySpacedRectSide\",\"uuid\":\"ea73d2ad-6043-4637-ba6c-414a87cf6777\"},{\"content\":{\"connectorIds\":[],\"side\":\"HIDDEN\"},\"type\":\"ConnectorPlacement.EquallySpacedRectSide\",\"uuid\":\"ed240fd2-007a-443e-85e9-b2acea2870c2\"}]},\"type\":\"ConnectorPlacement.EquallySpacedConnector\",\"uuid\":\"aa40401b-6e13-445e-a9b0-89ce19fbc40c\"}],\"packageUris\":[\"http://schema.mathworks.com/mf0/Connector/R2020b\"],\"version\":\"1.0\"}"
  Currents : Scope  NumInputPorts=2
  Demux : Demux  Outputs=2
  Demux1 : Demux  Outputs=2
  From6 : From  Commented=on  GotoTag=Iabc
  From7 : From  Commented=on  GotoTag=Vabc
  Meas_3_Wire : Subsystem
  Modulation : Scope  Commented=on
  Mux1 : Mux  Inputs=5
  Mux2 : Mux  Inputs=2
  Mux3 : Mux  Commented=on  Inputs=3
  "PMU (PLL-Based, Positive-Sequence)" : spsPMUPLLBasedPositiveSequenceLib/PMU (PLL-Based, Positive-Sequence)  Commented=on  nominalFrequency=60  samplingRate=48  reportingFactor=1
      settings: SourceProductBaseCode=PS
  "PMU (PLL-Based, Positive-Sequence)1" : spsPMUPLLBasedPositiveSequenceLib/PMU (PLL-Based, Positive-Sequence)  Commented=on  nominalFrequency=60  samplingRate=48  reportingFactor=1
      settings: SourceProductBaseCode=PS
  PMU_Current : Scope  Commented=on  NumInputPorts=3
  PMU_Voltage : Scope  Commented=on  NumInputPorts=3
  Park_Transformation : Subsystem
  Park_Transformation1 : Subsystem
  Power Control : Subsystem
      settings: PortSchema="{\"entries\":[{\"content\":{\"sides\":[{\"content\":{\"connectorIds\":[\"In1\"]},\"type\":\"ConnectorPlacement.EquallySpacedRectSide\",\"uuid\":\"974d39f2-3edd-4b06-9531-29f32c88933a\"},{\"content\":{\"connectorIds\":[\"Out1\"],\"side\":\"RIGHT\"},\"type\":\"ConnectorPlacement.EquallySpacedRectSide\",\"uuid\":\"24d62c8a-c61a-462a-84f0-1f0276c6dbaa\"},{\"content\":{\"connectorIds\":[],\"side\":\"TOP\"},\"type\":\"ConnectorPlacement.EquallySpacedRectSide\",\"uuid\":\"5ada6b1b-08a4-4e4d-9a20-cc19768e3a35\"},{\"content\":{\"connectorIds\":[\"In2\",\"In3\"],\"side\":\"BOTTOM\"},\"type\":\"ConnectorPlacement.EquallySpacedRectSide\",\"uuid\":\"aac35657-a4cf-4c82-a962-be637b231177\"},{\"content\":{\"connectorIds\":[],\"side\":\"HIDDEN\"},\"type\":\"ConnectorPlacement.EquallySpacedRectSide\",\"uuid\":\"6c2f95fb-9c8c-4eee-ad47-c57a643c3198\"}]},\"type\":\"ConnectorPlacement.EquallySpacedConnector\",\"uuid\":\"4f1b2c82-b884-470a-8be3-e486ca1ee764\"}],\"packageUris\":[\"http://schema.mathworks.com/mf0/Connector/R2020b\"],\"version\":\"1.0\"}"
  Power Measurement (Three-Phase) : eePowerMeasurement/Power Measurement (Three-Phase)  LabelModeActiveChoice=Discrete  F=60  K=[1]  Seq=Positive  Ts=Ts
      settings: SourceProductBaseCode=PS
  Product2 : Product
  SRF_PLL : Subsystem
  Saturation : Saturate  UpperLimit=1.1  LowerLimit=-1.1
  Terminator : Terminator
  Voltages : Scope  Commented=on  NumInputPorts=2
  Mabc : Outport
  Measures : Outport  Port=2
  Vabc : Outport  Port=3
  wires:
  SRF_PLL/1(Phase) -> [phase_pll]
  Park_Transformation/1(DQ) -> Currents/2, [Idq]
  [Vabc] -> SRF_PLL/1(Vabc)
  [Vabc] -> Voltages/1, Park_Transformation1/1(ABC)
  Park_Transformation1/1(DQ) -> Voltages/2, Demux1/1, [Vdq]
  [phase_pll] -> Park_Transformation1/2(Phase)
  Saturation/1 -> Mabc/1, Modulation/1
  [dblk] -> Product2/2
  Iabc/1 -> Park_Transformation/1(ABC), Currents/1, [Iabc]
  Meas_3_Wire/1(ABC) -> [Vabc]
  Product2/1 -> Saturation/1
  Vline/1 -> Demux/1
  Demux/1 -> Meas_3_Wire/1(AB)
  Demux/2 -> Meas_3_Wire/2(BC)
  Mux1/1 -> Measures/1
  [Vdq] -> Mux1/3
  [Iabc] -> Mux1/2
  [Vabc] -> Mux1/4, Vabc/1
  [Idq] -> Mux1/1
  From7/1 -> "PMU (PLL-Based, Positive-Sequence)"/1
  From6/1 -> "PMU (PLL-Based, Positive-Sequence)1"/1
  "PMU (PLL-Based, Positive-Sequence)"/1 -> PMU_Voltage/1
  "PMU (PLL-Based, Positive-Sequence)"/2 -> PMU_Voltage/2
  "PMU (PLL-Based, Positive-Sequence)"/3 -> PMU_Voltage/3
  "PMU (PLL-Based, Positive-Sequence)1"/1 -> Mux3/1, PMU_Current/1
  "PMU (PLL-Based, Positive-Sequence)1"/2 -> Mux3/2, PMU_Current/2
  "PMU (PLL-Based, Positive-Sequence)1"/3 -> Mux3/3, PMU_Current/3
  Deblock_inv/1 -> [dblk], Current Control/1(Deblock)
  Current Control/1(modulation) -> Product2/1
  [Idq] -> Current Control/3(Idq)
  [Vdq] -> Current Control/4(Vdq)
  [phase_pll] -> Current Control/5(Phase)
  [phase_pll] -> Park_Transformation/2(Phase)
  Demux1/2 -> Terminator/1
  Demux1/1 -> [Vd]
  PQ_ref/1 -> Power Control/1(PQ_ref)
  [Vd] -> Power Control/2(Vd)
  [dblk] -> Power Control/3(Dblk)
  Power Control/1(Out1) -> Current Control/2(Idq_ref)
  [Vabc] -> Power Measurement (Three-Phase)/1
  [Iabc] -> Power Measurement (Three-Phase)/2
  Power Measurement (Three-Phase)/2 -> Mux2/2
  Power Measurement (Three-Phase)/1 -> Mux2/1
  Mux2/1 -> [pq_meas]
  [pq_meas] -> Mux1/5

== system Basic_cosimulation_circuit/SM_Master/VSC_ITM_SFA/PWM ==
  Uabc_ref : Inport
  Constant10 : Constant  Value=2
  Constant11 : Constant  Value=fsw_inv
  Constant9 : Constant
  Demux8 : Demux  Outputs=3
  Divide7 : Product  Inputs=*/
  Divide8 : Product  Inputs=*/
  Divide9 : Product  Inputs=*/
  Mux11 : Mux  Inputs=3
  Mux12 : Mux  Inputs=2
  RTE Conversion1 : rteventslib/Signal Attributes/RTE Conversion  inputdatatype=RTE Boolean  outputdatatype=Double  compensation=Enabled  nbMaxEvents=4  sampleTime=Ts
  RTE SPWM1 : rteventslib/Sources/RTE SPWM  NumberPhases=3-ph  CenterAlignmentMode=On  MaxFreq=inf  MinFreq=0  EnablingPort=off  ComplementaryMode=on  SpaceVector=off  RiseTimeDelay=0  MaxEvents=4  SampleTime=Ts
  Scope : Scope
  Scope8 : Scope
  Selector1 : Selector  InputPortWidth=6  IndexOptions=Index vector (dialog)  Indices=[1 4 2 5 3 6]  OutputSizes=1
  Sum16 : Sum  Inputs=|++
  Sum17 : Sum  Inputs=|++
  Sum18 : Sum  Inputs=|++
  Uref : Outport  VectorParamsAs1DForOutWhenUnconnected=off
  wires:
  Uabc_ref/1 -> Demux8/1, Scope/1
  RTE SPWM1/1 -> Mux12/1
  Constant9/1 -> Sum18/2, Sum17/2, Sum16/2
  Selector1/1 -> Uref/1
  Constant11/1 -> RTE SPWM1/1
  Sum16/1 -> Divide7/1
  Constant10/1 -> Divide9/2, Divide8/2, Divide7/2
  Sum17/1 -> Divide8/1
  Divide9/1 -> Mux11/3
  RTE SPWM1/2 -> Mux12/2
  Demux8/2 -> Sum17/1
  Divide8/1 -> Mux11/2
  Sum18/1 -> Divide9/1
  Mux11/1 -> RTE SPWM1/2, Scope8/1
  Divide7/1 -> Mux11/1
  Demux8/1 -> Sum16/1
  Demux8/3 -> Sum18/1
  Mux12/1 -> RTE Conversion1/1
  RTE Conversion1/1 -> Selector1/1

== system Basic_cosimulation_circuit/SM_Master/VSC_ITM_SFA/Phasor_to_Time_Domain_SFA ==
  Dynamic_Phasor : Inport
  Complex to Real-Imag4 : ComplexToRealImag
  Constant : Constant  Value=offset
  Deg->Rad : Gain  Gain=pi/180
  Demux1 : Demux  Outputs=2
  Gain3 : Gain  Gain=2*pi
  Gain4 : Gain  Gain=j*1
  Integrator with Wrapped State (Discrete or Continuous) : eeGeneralControl/Integrator with Wrapped State (Discrete or Continuous)  LabelModeActiveChoice=Discrete  WrappedStateUpperValue=2*pi  WrappedStateLowerValue=0  x0=0  Ts=-1
      settings: SourceProductBaseCode=PS
  Magnitude-Angle to Complex : MagnitudeAngleToComplex
  Math Function : Math  SaturateOnIntegerOverflow=on
  Product : Product
  Terminator : Terminator
  EMT : Outport
  wires:
  Dynamic_Phasor/1 -> Demux1/1
  Product/1 -> Complex to Real-Imag4/1  "Analytic Signal"
  Magnitude-Angle to Complex/1 -> Product/1  "Dynamic Phasor"
  Complex to Real-Imag4/2 -> Terminator/1
  Complex to Real-Imag4/1 -> EMT/1
  Demux1/1 -> Magnitude-Angle to Complex/1
  Demux1/2 -> Deg->Rad/1
  Deg->Rad/1 -> Magnitude-Angle to Complex/2
  Constant/1 -> Gain3/1
  Math Function/1 -> Product/2  "Phase Shift"
  Gain4/1 -> Math Function/1
  Gain3/1 -> Integrator with Wrapped State (Discrete or Continuous)/1
  Integrator with Wrapped State (Discrete or Continuous)/1 -> Gain4/1

== system Basic_cosimulation_circuit/SM_Master/VSC_ITM_SFA/Three-Phase Controlled Y-Connected Voltage Source  ==
  Va : Inport
  Vb : Inport  Port=2
  Vc : Inport  Port=3
  Controlled Voltage Source : spsControlledVoltageSourceLib/Controlled Voltage Source  Initialize=on  Source_Type=AC  Amplitude=0  Phase=0  Frequency=0  Measurements=None
  Controlled Voltage Source1 : spsControlledVoltageSourceLib/Controlled Voltage Source  Initialize=on  Source_Type=AC  Amplitude=0  Phase=0  Frequency=0  Measurements=None
  Controlled Voltage Source2 : spsControlledVoltageSourceLib/Controlled Voltage Source  Initialize=on  Source_Type=AC  Amplitude=0  Phase=0  Frequency=0  Measurements=None
  Ground : spsGroundLib/Ground  LConnTagsString=a
  A : PMIOPort  Side=Right
  B : PMIOPort  Port=2  Side=Right
  C : PMIOPort  Port=3  Side=Right
  wires:
  Vb/1 -> Controlled Voltage Source1/1
  Va/1 -> Controlled Voltage Source/1
  Vc/1 -> Controlled Voltage Source2/1
  connections:
  Controlled Voltage Source/RConn1 -- A/RConn1
  Controlled Voltage Source1/RConn1 -- B/RConn1
  Controlled Voltage Source2/RConn1 -- C/RConn1
  Controlled Voltage Source2/LConn1 -- Controlled Voltage Source/LConn1 -- Controlled Voltage Source1/LConn1 -- Ground/LConn1

== system Basic_cosimulation_circuit/SM_Master/VSC_ITM_SFA/Time_Domain_To_Phasor_SFA ==
  EMT : Inport
  Complex to Magnitude-Angle : ComplexToMagnitudeAngle
  Frequency Offset : Constant  Value=offset
  Gain : Gain  Gain=j*(1/sqrt(3))*[0 1 -1; -1 0 1; 1 -1 0]  Multiplication=Matrix(K*u)
  Gain2 : Gain  Gain="[1  0 0; 0 1 0 ; 0 0 1]"  Multiplication=Matrix(K*u)
  Gain3 : Gain  Gain=2*pi
  Gain4 : Gain  Gain=j*-1
  Integrator with Wrapped State (Discrete or Continuous) : eeGeneralControl/Integrator with Wrapped State (Discrete or Continuous)  LabelModeActiveChoice=Discrete  WrappedStateUpperValue=2*pi  WrappedStateLowerValue=0  x0=0  Ts=-1
      settings: SourceProductBaseCode=PS
  Math Function : Math  SaturateOnIntegerOverflow=on
  Mux1 : Mux  Inputs=2
  Product : Product
  Rad->Deg : Gain  Gain=180/pi
  Sum1 : Sum  Inputs=+|+
  Dynamic_Phasor : Outport
  wires:
  Sum1/1 -> Product/1  "Analytic Signal"
  Mux1/1 -> Dynamic_Phasor/1
  Gain2/1 -> Sum1/2
  Complex to Magnitude-Angle/1 -> Mux1/1
  Gain/1 -> Sum1/1
  Rad->Deg/1 -> Mux1/2
  EMT/1 -> Gain/1, Gain2/1  "EMT Three-phase Signal"
  Product/1 -> Complex to Magnitude-Angle/1  "Dynamic Phasor"
  Complex to Magnitude-Angle/2 -> Rad->Deg/1
  Gain4/1 -> Math Function/1
  Frequency Offset/1 -> Gain3/1
  Math Function/1 -> Product/2  "Phase Shift"
  Gain3/1 -> Integrator with Wrapped State (Discrete or Continuous)/1
  Integrator with Wrapped State (Discrete or Continuous)/1 -> Gain4/1

== system Basic_cosimulation_circuit/SM_Master/Circuit_ITM_Source_DP_AW/DP - > EMT/Subsystem ==
  In1 : Inport
  Input : Inport  Port=2
  Compare To Constant : simulink/Logic and Bit Operations/Compare To Constant  relop=>=  const=2*pi  OutDataTypeStr=boolean
  Constant : Constant  Value=2*pi
  Constant2 : Constant  Value=2*pi*60
  Integrator : Integrator  ExternalReset=rising  InitialConditionSource=external  ShowStatePort=on
  Product4 : Product
  Sin3 : Trigonometry
  Sum : Sum  Inputs=|+-
  Sum4 : Sum  Inputs=|++
  Out1 : Outport
  wires:
  Product4/1 -> Out1/1
  In1/1 -> Product4/1
  Integrator/1 -> Sum4/2
  Input/1 -> Sum4/1
  Sum4/1 -> Sin3/1
  Sin3/1 -> Product4/2
  Integrator/State -> Sum/1, Compare To Constant/1
  Constant2/1 -> Integrator/1
  Compare To Constant/1 -> Integrator/2
  Sum/1 -> Integrator/3
  Constant/1 -> Sum/2

== system Basic_cosimulation_circuit/SM_Master/Circuit_ITM_Source_DP_AW/DP - > EMT/Subsystem1 ==
  In1 : Inport
  Input1 : Inport  Port=2
  Compare To Constant : simulink/Logic and Bit Operations/Compare To Constant  relop=>=  const=2*pi  OutDataTypeStr=boolean
  Constant : Constant  Value=2*pi
  Constant2 : Constant  Value=2*pi*60
  Integrator : Integrator  ExternalReset=rising  InitialConditionSource=external  ShowStatePort=on
  Product4 : Product
  Sin3 : Trigonometry
  Sum : Sum  Inputs=|+-
  Sum4 : Sum  Inputs=|++
  Out1 : Outport
  wires:
  Product4/1 -> Out1/1
  In1/1 -> Product4/1
  Integrator/1 -> Sum4/2
  Input1/1 -> Sum4/1
  Sum4/1 -> Sin3/1
  Sin3/1 -> Product4/2
  Constant/1 -> Sum/2
  Sum/1 -> Integrator/3
  Compare To Constant/1 -> Integrator/2
  Integrator/State -> Sum/1, Compare To Constant/1
  Constant2/1 -> Integrator/1

== system Basic_cosimulation_circuit/SM_Master/Circuit_ITM_Source_DP_AW/DP - > EMT/Subsystem2 ==
  In1 : Inport
  Input2 : Inport  Port=2
  Compare To Constant : simulink/Logic and Bit Operations/Compare To Constant  relop=>=  const=2*pi  OutDataTypeStr=boolean
  Constant : Constant  Value=2*pi
  Constant2 : Constant  Value=2*pi*60
  Integrator : Integrator  ExternalReset=rising  InitialConditionSource=external  ShowStatePort=on
  Product4 : Product
  Sin3 : Trigonometry
  Sum : Sum  Inputs=|+-
  Sum4 : Sum  Inputs=|++
  Out1 : Outport
  wires:
  Product4/1 -> Out1/1
  In1/1 -> Product4/1
  Integrator/1 -> Sum4/2
  Input2/1 -> Sum4/1
  Sum4/1 -> Sin3/1
  Sin3/1 -> Product4/2
  Integrator/State -> Sum/1, Compare To Constant/1
  Constant2/1 -> Integrator/1
  Compare To Constant/1 -> Integrator/2
  Sum/1 -> Integrator/3
  Constant/1 -> Sum/2
